simulink model "Zadatak2_antialiasing"  (R2020b)
settings: Solver=VariableStepAuto  StartTime=0.0  StopTime=10.0  RelTol=1e-3
libraries: dsparch4 x1
settings Model: Creator=user  LastModifiedBy=user

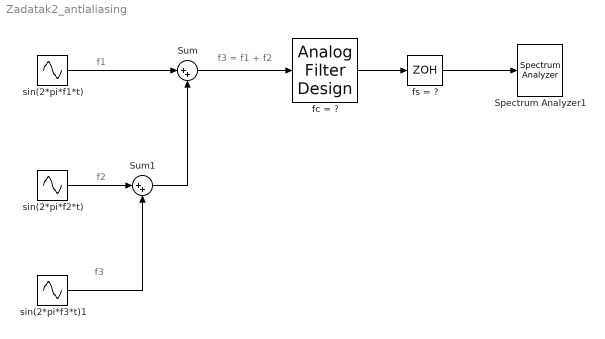
== system Zadatak2_antialiasing ==
  note: f3
  note: f2
  note: f1
  note: f3 = f1 + f2
  Spectrum Analyzer1 : SpectrumAnalyzer
  Sum : Sum  Inputs=|++
  Sum1 : Sum  Inputs=|++
  fc = ? : dsparch4/Analog Filter Design  method=Butterworth  filttype=Lowpass  N=8  Wlo=2*pi*200  Whi=2*pi*180  Rp=2  Rs=40
  fs = ? : ZeroOrderHold  SampleTime=0.0004
  sin(2*pi*f1*t) : Sin  Frequency=2*pi*100  SampleTime=0
  sin(2*pi*f2*t) : Sin  Frequency=2*pi*160  SampleTime=0
  sin(2*pi*f3*t)1 : Sin  Frequency=2*pi*1000  SampleTime=0
  wires:
  sin(2*pi*f1*t)/1 -> Sum/1
  sin(2*pi*f2*t)/1 -> Sum1/1
  Sum/1 -> fc = ?/1
  fc = ?/1 -> fs = ?/1
  fs = ?/1 -> Spectrum Analyzer1/1
  Sum1/1 -> Sum/2
  sin(2*pi*f3*t)1/1 -> Sum1/2
